simulink model "EMR_vehicle_model_EMRAX188"  (R2023a)
settings: Solver=VariableStepAuto  StartTime=0.0  StopTime=sim_time  RelTol=1e-3
values from neighbouring files (symbols this model uses):
  A_f = 2    [motor_parameters.m]
  air_dens = 1.22521    [motor_parameters.m]
  angle_road = atan(slope_road/100)    [motor_parameters.m]
  C_d = 0.35    [motor_parameters.m]
  converter_efficiency = 0.95    [motor_parameters.m]
  f_r = 0.017    [motor_parameters.m]
  g = 9.8    [motor_parameters.m]
  k_gear = 5    [motor_parameters.m]
  Kantiwind_d = Kp_current_d    [motor_parameters.m]
  Kantiwind_q = Kp_current_q    [motor_parameters.m]
  Ki_current_d = (log(9)/risingtime)*winding_resistance    [motor_parameters.m]
  Ki_current_q = (log(9)/risingtime)*winding_resistance    [motor_parameters.m]
  Kp_current_d = (log(9)/risingtime)*Ld    [motor_parameters.m]
  Kp_current_q = (log(9)/risingtime)*Lq    [motor_parameters.m]
  Kp_speed = m_v/tau_speed    (= 666.666666667)    [motor_parameters.m]
  lambdam = 0.072    [motor_parameters.m]
  Ld = 5.4e-6    (= 5.4e-06)    [motor_parameters.m]
  lower_current_limit = -upper_current_limit    (= -400)    [motor_parameters.m]
  lower_volt_limit = -upper_volt_limit    (= -110)    [motor_parameters.m]
  Lq = 6.0e-6    (= 6e-06)    [motor_parameters.m]
  m_v = 1000    [motor_parameters.m]
  polenumber = 2*polepairs    (= 20)    [motor_parameters.m]
  r_w = 0.26    [motor_parameters.m]
  Rbat = 0.1    [motor_parameters.m]
  upper_current_limit = 400    [motor_parameters.m]
  upper_volt_limit = 110    [motor_parameters.m]
  VDC = 800    [motor_parameters.m]
  wind_speed = 0    [motor_parameters.m]
  winding_resistance = 0.8e-3    (= 0.0008)    [motor_parameters.m]
libraries: simulink x2
settings Model: Creator=citcea  LastModifiedBy=citcea

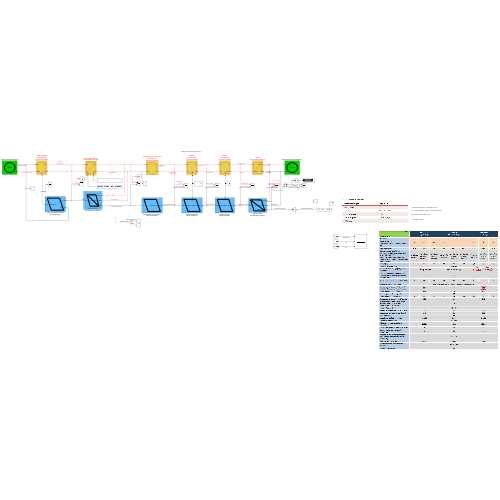
[thumbnail: Simulink's stored preview of the top-level diagram]
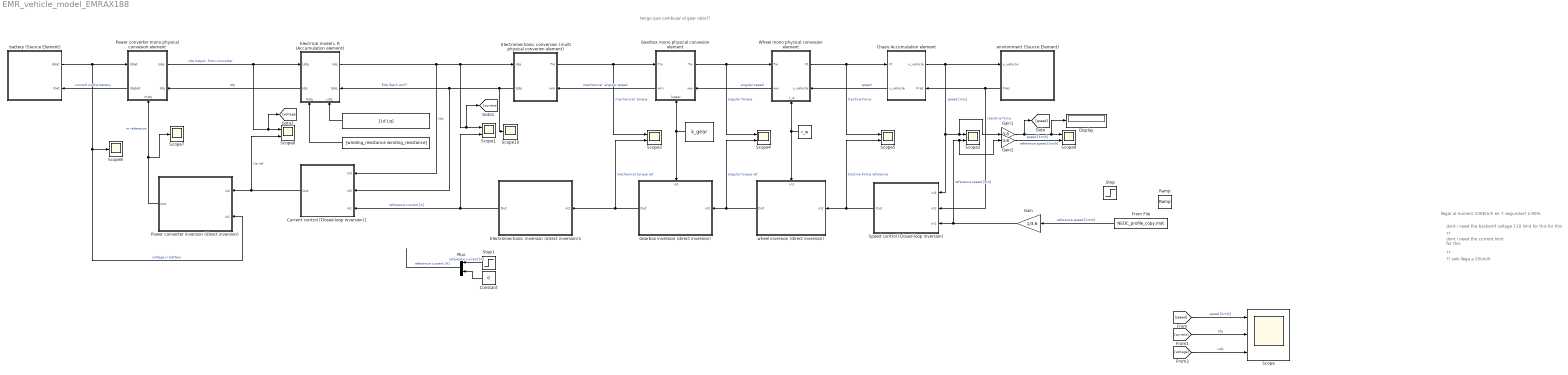
== system EMR_vehicle_model_EMRAX188 ==
  note: dont i need the current limit for this
  note: dont i need the backemf voltage 110 limit for this for this
  note: ?? solo llega a 35km/h
  note: ??
  note: ??
  note: llegar al numero 100Km/h en 7 segundos? o 90%
  note: tengo que cambuiar el gear ratio??
  " " : Constant  Value=[winding_resistance winding_resistance]
  "  " : Constant  Value=k_gear
  "   " : Constant  Value=[Ld Lq]
  "     " : Constant  Value=r_w
  Chasis Accumulation element : Subsystem  mask(CM){}
      settings: LibrarySourceBlock=simulink/REM/EA  PortSchema="{\"entries\":[{\"content\":{\"sides\":[{\"content\":{\"connectorIds\":[\"In1\",\"Out2\"]},\"type\":\"ConnectorPlacement.EquallySpacedRectSide\",\"uuid\":\"dba36025-b2f5-41cb-9761-d1287a9766e1\"},{\"content\":{\"connectorIds\":[\"Out1\",\"In2\"],\"side\":\"RIGHT\"},\"type\":\"ConnectorPlacement.EquallySpacedRectSide\",\"uuid\":\"3ae5e504-7b8f-4c00-bc0d-c89eccd87070\"},{\"content\":{\"side\":\"TOP\"},\"type\":\"ConnectorPlacement.EquallySpacedRectSide\",\"uuid\":\"a4c04bb5-f94e-4b5c-882d-2c32a11c6b0c\"}]},\"type\":\"ConnectorPlacement.EquallySpacedConnector\",\"uuid\":\"0c2b765b-f129-495b-87a6-76b6e14d78ec\"}],\"packageUris\":[\"http://schema.mathworks.com/mf0/Connector/R2020b\"],\"version\":\"1.0\"}"
      mask Display: plot(0,0,100,100,[10,10,90,90,10],[90,10,10,90,90], [10,90],[10,90])
  Constant : Constant  Value=0
  Current control (Closed-loop inversion)1 : Subsystem
      settings: LibrarySourceBlock=|
      | simulink/SMC/Asservissement
      | Correcteur IP
      mask Display: plot(0,0,100,100, [10,30,90,70,10,90],[90,10,10,90,90,10])
  Display : Display
  Electrical model L R (Accumulation element) : Subsystem  mask(CM){}
      settings: LibrarySourceBlock=simulink/REM/EA  PortSchema="{\"entries\":[{\"content\":{\"sides\":[{\"content\":{\"connectorIds\":[\"In1\",\"Out2\"]},\"type\":\"ConnectorPlacement.EquallySpacedRectSide\",\"uuid\":\"eb47d662-bb9b-4acd-af55-2a228b53d8b6\"},{\"content\":{\"connectorIds\":[\"Out1\",\"In4\"],\"side\":\"RIGHT\"},\"type\":\"ConnectorPlacement.EquallySpacedRectSide\",\"uuid\":\"c961b4fe-0170-40df-8b75-bfc3223dfb7e\"},{\"content\":{\"side\":\"TOP\"},\"type\":\"ConnectorPlacement.EquallySpacedRectSide\",\"uuid\":\"6474a77d-3f02-40ef-ac6e-8688b5dfe053\"},{\"content\":{\"connectorIds\":[\"In2\",\"In3\"],\"side\":\"BOTTOM\"},\"type\":\"ConnectorPlacement.EquallySpacedRectSide\",\"uuid\":\"8508c19b-50ed-4acb-b5ce-1a3d4ba68c03\"}]},\"type\":\"ConnectorPlacement.EquallySpacedConnector\",\"uuid\":\"ed0b028c-df9b-42ff-9675-f2eb8371642a\"}],\"packageUris\":[\"http://schema.mathworks.com/mf0/Connector/R2020b\"],\"version\":\"1.0\"}"
      mask Display: plot(0,0,100,100,[10,10,90,90,10],[90,10,10,90,90], [10,90],[10,90])
  Electromechanic conversion (multi physical converion element) : Subsystem
      settings: LibrarySourceBlock=simulink/REM/EC EM  PortSchema="{\"entries\":[{\"content\":{\"sides\":[{\"content\":{\"connectorIds\":[\"In1\",\"Out2\"]},\"type\":\"ConnectorPlacement.EquallySpacedRectSide\",\"uuid\":\"eb47d662-bb9b-4acd-af55-2a228b53d8b6\"},{\"content\":{\"connectorIds\":[\"Out1\",\"In2\"],\"side\":\"RIGHT\"},\"type\":\"ConnectorPlacement.EquallySpacedRectSide\",\"uuid\":\"c961b4fe-0170-40df-8b75-bfc3223dfb7e\"},{\"content\":{\"side\":\"TOP\"},\"type\":\"ConnectorPlacement.EquallySpacedRectSide\",\"uuid\":\"6474a77d-3f02-40ef-ac6e-8688b5dfe053\"},{\"content\":{\"side\":\"BOTTOM\"},\"type\":\"ConnectorPlacement.EquallySpacedRectSide\",\"uuid\":\"5fa3375e-1c74-4447-9856-dc04d4629517\"}]},\"type\":\"ConnectorPlacement.EquallySpacedConnector\",\"uuid\":\"ed0b028c-df9b-42ff-9675-f2eb8371642a\"}],\"packageUris\":[\"http://schema.mathworks.com/mf0/Connector/R2020b\"],\"version\":\"1.0\"}"
      mask Display: plot(0,0,100,100, 1.4*[50,57.68,60.77,63.08,64.97,66.58,68,69.26,70.4, 	71.42,72.36,78.28,80,78.28,72.36,71.42,70.4, 	69.26,68,66.58,64.97,63.08,60.77,57.68,50,42.32, 	39.23,36.92,35.03,33.42,32,30.74,29.6,28.58, 	27.64,21.72,20,21.72,27.64,28.58,29.6,30.74,32, 	33.42,35.03,36.92,39.23,42.32,50]-20, 1.4*[20,21,22,23,24,25,26,27,28,29,30,40,50,60,70,71,72, 	73,74,75,76,77,78,79,80,79,78,77,76,75,74,73,72, 	71,70,60,50,40,30,29,28,27,26,25,24,23,22,21,20]-20)
  Electromechanic inversion (direct inversion)1 : Subsystem
      settings: LibrarySourceBlock=|
      | simulink/SMC/Inversion EC
      | avec mesure
      mask Display: plot(0,0,100,100,[10,30,90,70,10],[90,10,10,90,90])
  From File : FromFile  FileName=NEDC_profile_copy.mat  SampleTime=0
  Gain : Gain  Gain=1/3.6
  Gain1 : Gain  Gain=3.6
  Gain2 : Gain  Gain=3.6
  Gearbox mono physical convesion element : Subsystem  mask(Hacheur){}
      settings: LibrarySourceBlock=simulink/REM/EC Elec  PortSchema="{\"entries\":[{\"content\":{\"sides\":[{\"content\":{\"connectorIds\":[\"In1\",\"Out2\"]},\"type\":\"ConnectorPlacement.EquallySpacedRectSide\",\"uuid\":\"add9fadb-0fb4-43ab-a2d0-7727804eb2c0\"},{\"content\":{\"connectorIds\":[\"Out1\",\"In3\"],\"side\":\"RIGHT\"},\"type\":\"ConnectorPlacement.EquallySpacedRectSide\",\"uuid\":\"87b3f5c0-7da9-421a-ae8a-66afee038ab7\"},{\"content\":{\"side\":\"TOP\"},\"type\":\"ConnectorPlacement.EquallySpacedRectSide\",\"uuid\":\"1a4f8f42-25ac-452e-8ff7-6a9f16bc9892\"},{\"content\":{\"connectorIds\":[\"In2\"],\"side\":\"BOTTOM\"},\"type\":\"ConnectorPlacement.EquallySpacedRectSide\",\"uuid\":\"62447f74-8a92-4f32-9436-8aa69c6390a6\"}]},\"type\":\"ConnectorPlacement.EquallySpacedConnector\",\"uuid\":\"bc965109-6171-440e-b0fd-d7c986fb98ff\"}],\"packageUris\":[\"http://schema.mathworks.com/mf0/Connector/R2020b\"],\"version\":\"1.0\"}"
      mask Display: plot(0,0,100,100,[10,10,90,90,10],[90,10,10,90,90])
  Gearbox inversion (direct inversion) : Subsystem
      settings: PortSchema="{\"entries\":[{\"content\":{\"sides\":[{\"content\":{\"connectorIds\":[\"In1\"]},\"type\":\"ConnectorPlacement.EquallySpacedRectSide\",\"uuid\":\"89460601-ef91-4e28-89d9-1739ebd446c6\"},{\"content\":{\"connectorIds\":[\"Out1\"],\"side\":\"RIGHT\"},\"type\":\"ConnectorPlacement.EquallySpacedRectSide\",\"uuid\":\"1ce34b6b-3a45-4c28-907b-ce0af421135c\"},{\"content\":{\"connectorIds\":[\"In2\"],\"side\":\"TOP\"},\"type\":\"ConnectorPlacement.EquallySpacedRectSide\",\"uuid\":\"71132fa1-5c16-4a2a-8ec5-329f0796b3f7\"}]},\"type\":\"ConnectorPlacement.EquallySpacedConnector\",\"uuid\":\"f923a9d4-f6d6-49f7-92ef-115028220a52\"}],\"packageUris\":[\"http://schema.mathworks.com/mf0/Connector/R2020b\"],\"version\":\"1.0\"}"
      settings: LibrarySourceBlock=|
      | simulink/SMC/Inversion EC
      | avec mesure
      mask Display: plot(0,0,100,100,[10,30,90,70,10],[90,10,10,90,90])
  Mux : Mux  Inputs=2
  Power converter mono physical convesion element : Subsystem  mask(Hacheur){}
      settings: LibrarySourceBlock=simulink/REM/EC Elec  PortSchema="{\"entries\":[{\"content\":{\"sides\":[{\"content\":{\"connectorIds\":[\"In1\",\"Out2\"]},\"type\":\"ConnectorPlacement.EquallySpacedRectSide\",\"uuid\":\"add9fadb-0fb4-43ab-a2d0-7727804eb2c0\"},{\"content\":{\"connectorIds\":[\"Out1\",\"In3\"],\"side\":\"RIGHT\"},\"type\":\"ConnectorPlacement.EquallySpacedRectSide\",\"uuid\":\"87b3f5c0-7da9-421a-ae8a-66afee038ab7\"},{\"content\":{\"side\":\"TOP\"},\"type\":\"ConnectorPlacement.EquallySpacedRectSide\",\"uuid\":\"1a4f8f42-25ac-452e-8ff7-6a9f16bc9892\"},{\"content\":{\"connectorIds\":[\"In2\"],\"side\":\"BOTTOM\"},\"type\":\"ConnectorPlacement.EquallySpacedRectSide\",\"uuid\":\"62447f74-8a92-4f32-9436-8aa69c6390a6\"}]},\"type\":\"ConnectorPlacement.EquallySpacedConnector\",\"uuid\":\"bc965109-6171-440e-b0fd-d7c986fb98ff\"}],\"packageUris\":[\"http://schema.mathworks.com/mf0/Connector/R2020b\"],\"version\":\"1.0\"}"
      mask Display: plot(0,0,100,100,[10,10,90,90,10],[90,10,10,90,90])
  Power converter inversion (direct inversion) : Subsystem
      settings: LibrarySourceBlock=|
      | simulink/SMC/Inversion EC
      | avec mesure
      mask Display: plot(0,0,100,100,[10,30,90,70,10],[90,10,10,90,90])
  Ramp : simulink/Sources/Ramp  slope=100/7  start=0  InitialOutput=0
  Scope : Scope  NumInputPorts=3
  Scope{1..6,9} (7 alike) : Scope  NumInputPorts=2
  Scope10 : Scope
  Scope7 : Scope
  Scope8 : Scope
  Speed control (Closed-loop inversion) : Subsystem
      settings: LibrarySourceBlock=|
      | simulink/SMC/Asservissement
      | Correcteur IP
      mask Display: plot(0,0,100,100, [10,30,90,70,10,90],[90,10,10,90,90,10])
  Step : Step  After=120  SampleTime=0
  Step1 : Step  Time=0  After=100  SampleTime=0
  Wheel mono physical convesion element : Subsystem  mask(Hacheur){}
      settings: LibrarySourceBlock=simulink/REM/EC Elec  PortSchema="{\"entries\":[{\"content\":{\"sides\":[{\"content\":{\"connectorIds\":[\"In1\",\"Out2\"]},\"type\":\"ConnectorPlacement.EquallySpacedRectSide\",\"uuid\":\"add9fadb-0fb4-43ab-a2d0-7727804eb2c0\"},{\"content\":{\"connectorIds\":[\"Out1\",\"In3\"],\"side\":\"RIGHT\"},\"type\":\"ConnectorPlacement.EquallySpacedRectSide\",\"uuid\":\"87b3f5c0-7da9-421a-ae8a-66afee038ab7\"},{\"content\":{\"side\":\"TOP\"},\"type\":\"ConnectorPlacement.EquallySpacedRectSide\",\"uuid\":\"1a4f8f42-25ac-452e-8ff7-6a9f16bc9892\"},{\"content\":{\"connectorIds\":[\"In2\"],\"side\":\"BOTTOM\"},\"type\":\"ConnectorPlacement.EquallySpacedRectSide\",\"uuid\":\"cb138da9-d7db-4398-93fc-4ebc55a3031f\"}]},\"type\":\"ConnectorPlacement.EquallySpacedConnector\",\"uuid\":\"bc965109-6171-440e-b0fd-d7c986fb98ff\"}],\"packageUris\":[\"http://schema.mathworks.com/mf0/Connector/R2020b\"],\"version\":\"1.0\"}"
      mask Display: plot(0,0,100,100,[10,10,90,90,10],[90,10,10,90,90])
  battery (Source Element) : Subsystem
      settings: LibrarySourceBlock=simulink/REM/SE  PortSchema="{\"entries\":[{\"content\":{\"sides\":[{\"content\":{\"connectorIds\":[\"In1\",\"Out1\"]},\"type\":\"ConnectorPlacement.EquallySpacedRectSide\",\"uuid\":\"5172ac9f-d5c1-4cd8-b96a-59474b42a5b1\"},{\"content\":{\"side\":\"RIGHT\"},\"type\":\"ConnectorPlacement.EquallySpacedRectSide\",\"uuid\":\"2f1e5561-012a-4a4f-9618-a2ea7815b4bb\"},{\"content\":{\"side\":\"TOP\"},\"type\":\"ConnectorPlacement.EquallySpacedRectSide\",\"uuid\":\"04863bbd-e2a6-484f-917f-c8a12d5dbdba\"}]},\"type\":\"ConnectorPlacement.EquallySpacedConnector\",\"uuid\":\"d1a021b9-616a-4321-9b00-fb5e0223e97f\"}],\"packageUris\":[\"http://schema.mathworks.com/mf0/Connector/R2020b\"],\"version\":\"1.0\"}"
      mask Display:
      | plot(0,0,100,100, 1.2*[50,57.68,60.77,63.08,64.97,66.58,68,69.26,70.4, 	71.42,72.36,78.28,80,78.28,72.36,71.42,70.4, 	69.26,68,66.58,64.97,63.08,60.77,57.68,50,42.32, 	39.23,36.92,35.03,33.42,32,30.74,29.6,28.58, 	27.64,21.72,20,21.72,27.64,28.58,29.6,30.74,32, 	33.42,35.03,36.92,39.23,42.32,50]-10, 1.2*[20,21,22,23,24,25,26,27,28,29,30,40,50,60,70,71,72, 	73,74,75,76,77,78,79,80,79,78,77,76,75,74,73,72, 	71,70,60,50,40,30,29,28,27,26,25,24,23,22,21,20]-10)
      | disp('Source')
  environment (Source Element) : Subsystem
      settings: LibrarySourceBlock=simulink/REM/SE  PortSchema="{\"entries\":[{\"content\":{\"sides\":[{\"content\":{\"connectorIds\":[\"In1\",\"Out1\"]},\"type\":\"ConnectorPlacement.EquallySpacedRectSide\",\"uuid\":\"5172ac9f-d5c1-4cd8-b96a-59474b42a5b1\"},{\"content\":{\"side\":\"RIGHT\"},\"type\":\"ConnectorPlacement.EquallySpacedRectSide\",\"uuid\":\"2f1e5561-012a-4a4f-9618-a2ea7815b4bb\"},{\"content\":{\"side\":\"TOP\"},\"type\":\"ConnectorPlacement.EquallySpacedRectSide\",\"uuid\":\"04863bbd-e2a6-484f-917f-c8a12d5dbdba\"}]},\"type\":\"ConnectorPlacement.EquallySpacedConnector\",\"uuid\":\"d1a021b9-616a-4321-9b00-fb5e0223e97f\"}],\"packageUris\":[\"http://schema.mathworks.com/mf0/Connector/R2020b\"],\"version\":\"1.0\"}"
      mask Display:
      | plot(0,0,100,100, 1.2*[50,57.68,60.77,63.08,64.97,66.58,68,69.26,70.4, 	71.42,72.36,78.28,80,78.28,72.36,71.42,70.4, 	69.26,68,66.58,64.97,63.08,60.77,57.68,50,42.32, 	39.23,36.92,35.03,33.42,32,30.74,29.6,28.58, 	27.64,21.72,20,21.72,27.64,28.58,29.6,30.74,32, 	33.42,35.03,36.92,39.23,42.32,50]-10, 1.2*[20,21,22,23,24,25,26,27,28,29,30,40,50,60,70,71,72, 	73,74,75,76,77,78,79,80,79,78,77,76,75,74,73,72, 	71,70,60,50,40,30,29,28,27,26,25,24,23,22,21,20]-10)
      | disp('Source')
  wheel inversion (direct inversion) : Subsystem
      settings: PortSchema="{\"entries\":[{\"content\":{\"sides\":[{\"content\":{\"connectorIds\":[\"In1\"]},\"type\":\"ConnectorPlacement.EquallySpacedRectSide\",\"uuid\":\"89460601-ef91-4e28-89d9-1739ebd446c6\"},{\"content\":{\"connectorIds\":[\"Out1\"],\"side\":\"RIGHT\"},\"type\":\"ConnectorPlacement.EquallySpacedRectSide\",\"uuid\":\"1ce34b6b-3a45-4c28-907b-ce0af421135c\"},{\"content\":{\"connectorIds\":[\"In2\"],\"side\":\"TOP\"},\"type\":\"ConnectorPlacement.EquallySpacedRectSide\",\"uuid\":\"71132fa1-5c16-4a2a-8ec5-329f0796b3f7\"}]},\"type\":\"ConnectorPlacement.EquallySpacedConnector\",\"uuid\":\"f923a9d4-f6d6-49f7-92ef-115028220a52\"}],\"packageUris\":[\"http://schema.mathworks.com/mf0/Connector/R2020b\"],\"version\":\"1.0\"}"
      settings: LibrarySourceBlock=|
      | simulink/SMC/Inversion EC
      | avec mesure
      mask Display: plot(0,0,100,100,[10,30,90,70,10],[90,10,10,90,90])
  wires:
  environment (Source Element)/1(Fres) -> Chasis Accumulation element/2(Fres), Speed control (Closed-loop inversion)/2(in2)  "resistive force"
  Speed control (Closed-loop inversion)/1(Out) -> Scope5/2, wheel inversion (direct inversion)/1(in2)  "tractive Force reference"
  Chasis Accumulation element/2(v_vehicle) -> Wheel mono physical convesion element/3(v_vehicle)  "speed"
  "     "/1 -> Wheel mono physical convesion element/2(r_w), wheel inversion (direct inversion)/2(in1)
  Gearbox mono physical convesion element/1("Tw ") -> Scope4/1, Wheel mono physical convesion element/1(Tw)  "angular Torque"
  Wheel mono physical convesion element/2(ww) -> Gearbox mono physical convesion element/3(ww)  "angular speed"
  "  "/1 -> Gearbox inversion (direct inversion)/2(in1), Gearbox mono physical convesion element/2(kgear)
  Electromechanic conversion (multi physical converion element)/1("Tm ") -> Scope3/1, Gearbox mono physical convesion element/1(Tm)  "mechanical  torque"
  Gearbox mono physical convesion element/2(wm) -> Electromechanic conversion (multi physical converion element)/2(wm)  "mechanical  angular speed"
  Electrical model L R (Accumulation element)/1("Idq ") -> Current control (Closed-loop inversion)1/1(in3), [current], Scope1/1, Electromechanic conversion (multi physical converion element)/1(Idq)  "Idq"
  Electromechanic conversion (multi physical converion element)/2(Edq) -> Scope10/1, Current control (Closed-loop inversion)1/2(in5), Electrical model L R (Accumulation element)/4(Edq)  "Edq (back emf)"
  Electrical model L R (Accumulation element)/2(Idq) -> Power converter mono physical convesion element/3(Idq)  "Idq"
  Power converter mono physical convesion element/1("Udq ") -> Electrical model L R (Accumulation element)/1(Udq), [voltage], Scope6/1  "vdq output  from converter"
  Power converter mono physical convesion element/2("Idqbat  ") -> battery (Source Element)/1(Ibat)  "current on the battery"
  battery (Source Element)/1(Ubat) -> Power converter inversion (direct inversion)/2(in1), Scope8/1, Power converter mono physical convesion element/1(Ubat)  "voltage in battery"
  " "/1 -> Electrical model L R (Accumulation element)/2(Rdq)
  "   "/1 -> Electrical model L R (Accumulation element)/3(Ldq)
  Chasis Accumulation element/1("v_vehicle ") -> Speed control (Closed-loop inversion)/1(in3), Gain1/1, Scope2/1, environment (Source Element)/1(v_vehicle)  "speed [m/s]"
  wheel inversion (direct inversion)/1(Out) -> Gearbox inversion (direct inversion)/1(in2), Scope4/2  "angular torque ref"
  Gearbox inversion (direct inversion)/1(Out) -> Scope3/2, Electromechanic inversion (direct inversion)1/1(in2)  "mechanical torque ref"
  Current control (Closed-loop inversion)1/1(Out) -> Scope6/2, Power converter inversion (direct inversion)/1(in2)  "Ua ref"
  Power converter inversion (direct inversion)/1(Out) -> Scope7/1, Power converter mono physical convesion element/2(mdq)  "m reference"
  Gain/1 -> Gain2/1, Scope2/2, Speed control (Closed-loop inversion)/3(in1)  "reference speed [m/s]"
  From File/1 -> Gain/1  "reference speed [km/h]"
  Gain2/1 -> Scope9/2  "reference speed [km/h]"
  Gain1/1 -> [speed], Display/1, Scope9/1  "speed [km/h]"
  Electromechanic inversion (direct inversion)1/1(Out) -> Current control (Closed-loop inversion)1/3(in1), Scope1/2  "reference current [A]"
  Wheel mono physical convesion element/1("Ft ") -> Chasis Accumulation element/1(Ft), Scope5/1  "tractive Force"
  Step1/1 -> Mux/1  "reference current [A]"
  Constant/1 -> Mux/2
  Mux/1 -> ?  "reference current [A]"
  [speed] -> Scope/1  "speed [km/h]"
  [current] -> Scope/2  "Idq"
  [voltage] -> Scope/3  "vdq"

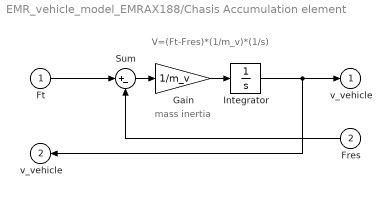
== system EMR_vehicle_model_EMRAX188/Chasis Accumulation element ==
  note: V=(Ft-Fres)*(1/m_v)*(1/s)
  note: mass inertia
  Ft : Inport
  Fres : Inport  Port=2
  Gain : Gain  Gain=1/m_v
  Integrator : Integrator
  Sum : Sum  Inputs=|+-
  "v_vehicle " : Outport  InitialOutput=0
  v_vehicle : Outport  Port=2  InitialOutput=0
  wires:
  Gain/1 -> Integrator/1
  Sum/1 -> Gain/1
  Integrator/1 -> v_vehicle/1, "v_vehicle "/1
  Ft/1 -> Sum/1
  Fres/1 -> Sum/2

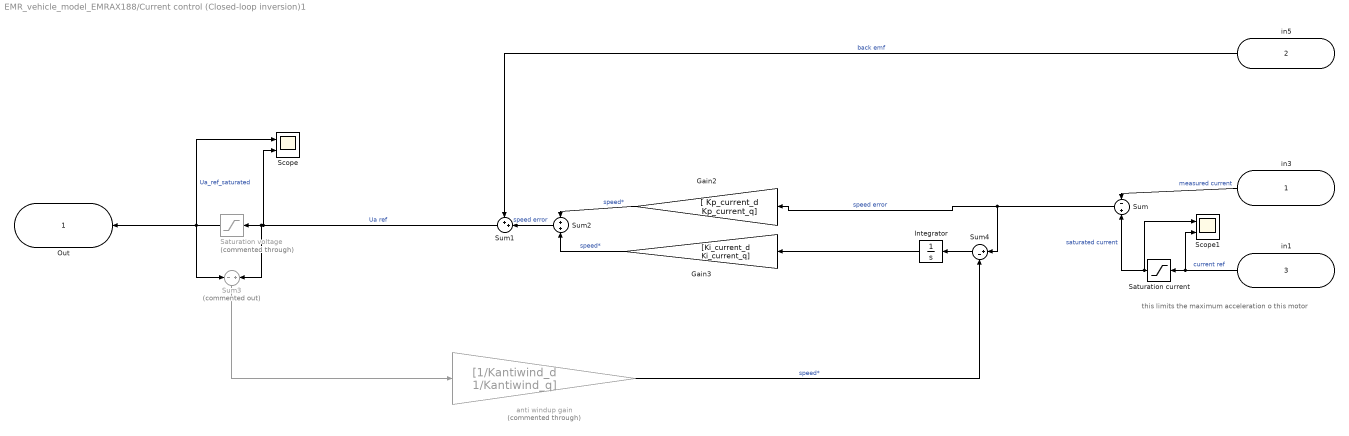
== system EMR_vehicle_model_EMRAX188/Current control (Closed-loop inversion)1 ==
  note: this limits the maximum acceleration o this motor
  in3 : Inport
  in5 : Inport  Port=2
  in1 : Inport  Port=3
  Gain2 : Gain  Gain=[ Kp_current_d Kp_current_q]
  Gain3 : Gain  Gain=[Ki_current_d Ki_current_q]
  Integrator : Integrator
  Saturation current : Saturate  UpperLimit=upper_current_limit  LowerLimit=lower_current_limit
  Saturation voltage : Saturate  Commented=through  UpperLimit=upper_volt_limit  LowerLimit=lower_volt_limit
  Scope : Scope  NumInputPorts=2
  Scope1 : Scope  NumInputPorts=2
  Sum : Sum  Inputs=-+
  Sum1 : Sum  Inputs=++|
  Sum2 : Sum
  Sum3 : Sum  Commented=on  Inputs=-|+
  Sum4 : Sum  Inputs=|+-
  anti windup gain : Gain  Commented=through  Gain=[1/Kantiwind_d 1/Kantiwind_q]
  Out : Outport  InitialOutput=0
  wires:
  in3/1 -> Sum/1  "measured current"
  in1/1 -> Scope1/2, Saturation current/1  "current ref"
  Sum1/1 -> Sum3/2, Saturation voltage/1, Scope/2  "Ua ref"
  Sum/1 -> Gain2/1, Sum4/1  "speed error"
  Gain2/1 -> Sum2/1  "speed*"
  in5/1 -> Sum1/1  "back emf"
  Gain3/1 -> Sum2/2  "speed*"
  Sum2/1 -> Sum1/2  "speed error"
  Integrator/1 -> Gain3/1
  Saturation current/1 -> Sum/2, Scope1/1  "saturated current"
  Saturation voltage/1 -> Sum3/1, Scope/1, Out/1  "Ua_ref_saturated"
  Sum3/1 -> anti windup gain/1
  anti windup gain/1 -> Sum4/2  "speed*"
  Sum4/1 -> Integrator/1

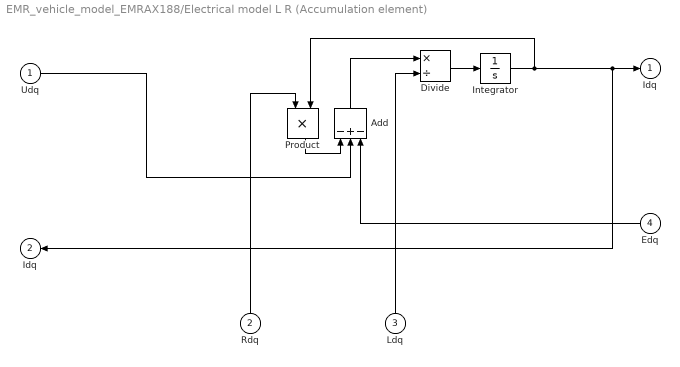
== system EMR_vehicle_model_EMRAX188/Electrical model L R (Accumulation element) ==
  Udq : Inport
  Rdq : Inport  Port=2
  Ldq : Inport  Port=3
  Edq : Inport  Port=4
  Add : Sum  Inputs=-+-
  Divide : Product  Inputs=*/
  Integrator : Integrator
  Product : Product
  "Idq " : Outport  InitialOutput=0
  Idq : Outport  Port=2  InitialOutput=0
  wires:
  Edq/1 -> Add/3
  Udq/1 -> Add/2
  Integrator/1 -> Product/2, "Idq "/1, Idq/1
  Add/1 -> Divide/1
  Ldq/1 -> Divide/2
  Divide/1 -> Integrator/1
  Product/1 -> Add/1
  Rdq/1 -> Product/1

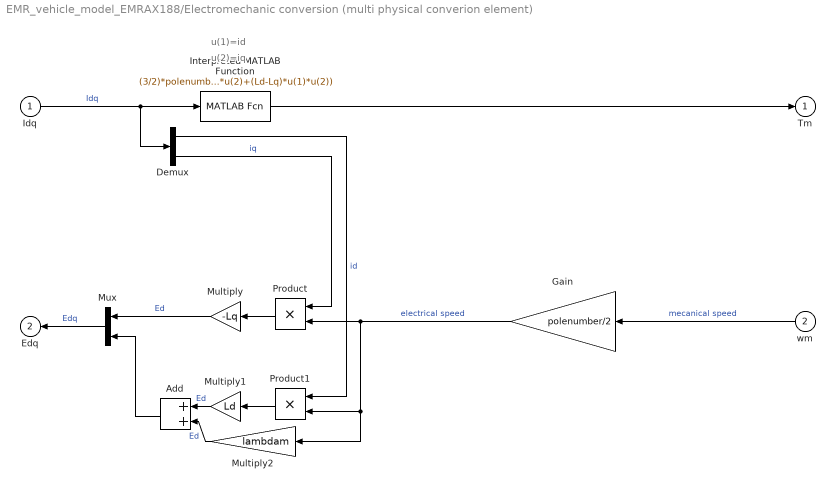
== system EMR_vehicle_model_EMRAX188/Electromechanic conversion (multi physical converion element) ==
  note: u(1)=id
  note: u(2)=iq
  Idq : Inport
  wm : Inport  Port=2
  Add : Sum
  Demux : Demux  Outputs=2
  Gain : Gain  Gain=polenumber/2
  Interpreted MATLAB Function : MATLABFcn  MATLABFcn=(3/2)*polenumber/2*(lambdam*u(2)+(Ld-Lq)*u(1)*u(2))  OutputDimensions=1
  Multiply : Gain  Gain=-Lq
  Multiply1 : Gain  Gain=Ld
  Multiply2 : Gain  Gain=lambdam
  Mux : Mux  Inputs=2
  Product : Product
  Product1 : Product
  "Tm " : Outport  InitialOutput=0
  Edq : Outport  Port=2  InitialOutput=0
  wires:
  Idq/1 -> Demux/1, Interpreted MATLAB Function/1  "Idq"
  Interpreted MATLAB Function/1 -> "Tm "/1
  wm/1 -> Gain/1  "mecanical speed"
  Demux/1 -> Product1/1  "id"
  Demux/2 -> Product/1  "iq"
  Mux/1 -> Edq/1  "Edq"
  Gain/1 -> Multiply2/1, Product1/2, Product/2  "electrical speed"
  Product/1 -> Multiply/1
  Multiply/1 -> Mux/1  "Ed"
  Product1/1 -> Multiply1/1
  Multiply1/1 -> Add/1  "Ed"
  Add/1 -> Mux/2
  Multiply2/1 -> Add/2  "Ed"

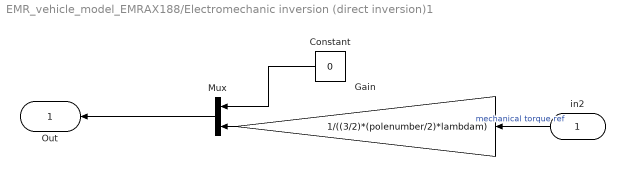
== system EMR_vehicle_model_EMRAX188/Electromechanic inversion (direct inversion)1 ==
  in2 : Inport
  Constant : Constant  Value=0
  Gain : Gain  Gain=1/((3/2)*(polenumber/2)*lambdam)
  Mux : Mux  Inputs=2
  Out : Outport  InitialOutput=0
  wires:
  Mux/1 -> Out/1
  Gain/1 -> Mux/2
  in2/1 -> Gain/1  "mechanical torque ref"
  Constant/1 -> Mux/1

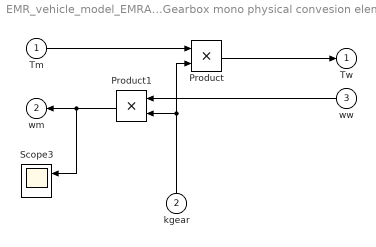
== system EMR_vehicle_model_EMRAX188/Gearbox mono physical convesion element ==
  Tm : Inport
  kgear : Inport  Port=2
  ww : Inport  Port=3
  Product : Product
  Product1 : Product
  Scope3 : Scope  NumInputPorts=2
  "Tw " : Outport  InitialOutput=0
  wm : Outport  Port=2  InitialOutput=0
  wires:
  Product1/1 -> Scope3/1, wm/1
  kgear/1 -> Product1/2, Product/2
  ww/1 -> Product1/1
  Product/1 -> "Tw "/1
  Tm/1 -> Product/1

== system EMR_vehicle_model_EMRAX188/Gearbox inversion (direct inversion) ==
  in2 : Inport
  in1 : Inport  Port=2
  Divide : Product  Inputs=/*
  Out : Outport  InitialOutput=0
  wires:
  Divide/1 -> Out/1  "mecanical torque"
  in2/1 -> Divide/2  "angular torque ref"
  in1/1 -> Divide/1  "k gear"

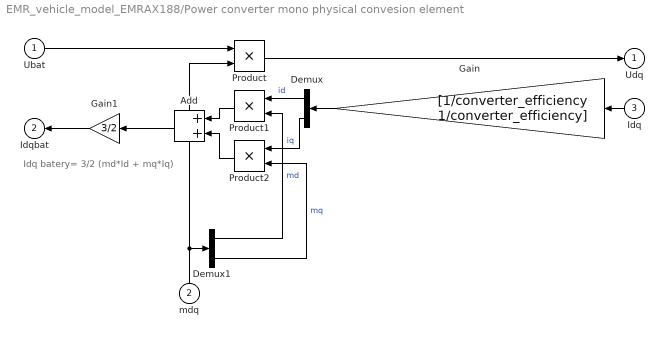
== system EMR_vehicle_model_EMRAX188/Power converter mono physical convesion element ==
  note: Idq batery= 3/2 (md*Id + mq*Iq)
  Ubat : Inport
  mdq : Inport  Port=2
  Idq : Inport  Port=3
  Add : Sum
  Demux : Demux  Outputs=2
  Demux1 : Demux  Outputs=2
  Gain : Gain  Gain=[1/converter_efficiency 1/converter_efficiency]
  Gain1 : Gain  Gain=3/2
  Product : Product
  Product1 : Product
  Product2 : Product
  "Udq " : Outport  InitialOutput=0
  "Idqbat  " : Outport  Port=2  InitialOutput=0
  wires:
  Idq/1 -> Gain/1
  Ubat/1 -> Product/1
  mdq/1 -> Demux1/1, Product/2
  Product/1 -> "Udq "/1
  Gain/1 -> Demux/1
  Gain1/1 -> "Idqbat  "/1
  Demux/1 -> Product1/1  "id"
  Demux/2 -> Product2/1  "iq"
  Demux1/1 -> Product1/2  "md"
  Demux1/2 -> Product2/2  "mq"
  Product1/1 -> Add/1
  Product2/1 -> Add/2
  Add/1 -> Gain1/1

== system EMR_vehicle_model_EMRAX188/Power converter inversion (direct inversion) ==
  in2 : Inport
  in1 : Inport  Port=2
  Divide : Product  Inputs=/*
  Saturation m ( we got regenerative braking) : Saturate  UpperLimit=1  LowerLimit=-1
  Out : Outport  InitialOutput=0
  wires:
  Divide/1 -> Saturation m ( we got regenerative braking)/1  "m_not saturated"
  in2/1 -> Divide/2  "Ua_dq ref"
  in1/1 -> Divide/1  "Ubat_dq"
  Saturation m ( we got regenerative braking)/1 -> Out/1  "mdq_ref_saturated"

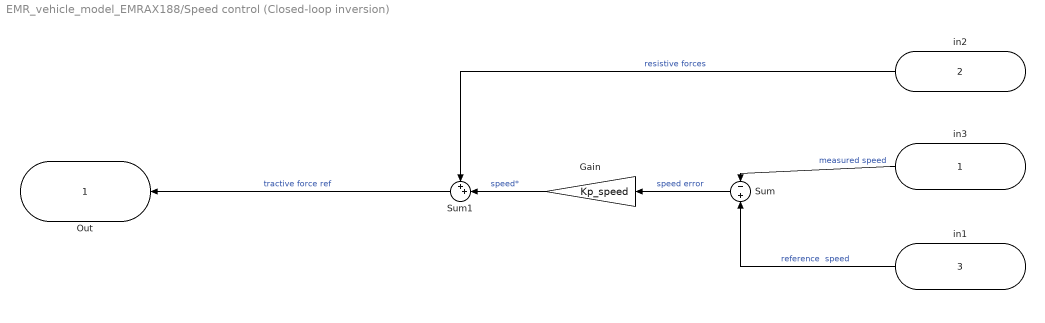
== system EMR_vehicle_model_EMRAX188/Speed control (Closed-loop inversion) ==
  in3 : Inport
  in2 : Inport  Port=2
  in1 : Inport  Port=3
  Gain : Gain  Gain=Kp_speed
  Sum : Sum  Inputs=-+
  Sum1 : Sum  Inputs=++|
  Out : Outport  InitialOutput=0
  wires:
  in3/1 -> Sum/1  "measured speed"
  in1/1 -> Sum/2  "reference  speed"
  Sum1/1 -> Out/1  "tractive force ref"
  Sum/1 -> Gain/1  "speed error"
  Gain/1 -> Sum1/2  "speed*"
  in2/1 -> Sum1/1  "resistive forces"

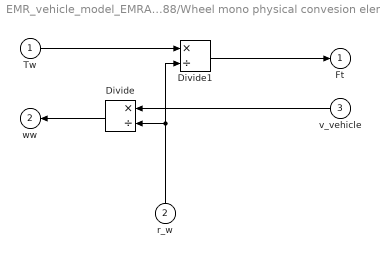
== system EMR_vehicle_model_EMRAX188/Wheel mono physical convesion element ==
  Tw : Inport
  r_w : Inport  Port=2
  v_vehicle : Inport  Port=3
  Divide : Product  Inputs=*/
  Divide1 : Product  Inputs=*/
  "Ft " : Outport  InitialOutput=0
  ww : Outport  Port=2  InitialOutput=0
  wires:
  Divide/1 -> ww/1
  v_vehicle/1 -> Divide/1
  r_w/1 -> Divide1/2, Divide/2
  Divide1/1 -> "Ft "/1
  Tw/1 -> Divide1/1

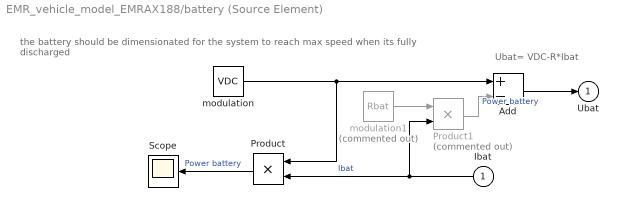
== system EMR_vehicle_model_EMRAX188/battery (Source Element) ==
  note: the battery should be dimensionated for the system to reach
      | max speed when its fully discharged
  note: Ubat= VDC-R*Ibat
  Ibat : Inport
  Add : Sum  Inputs=+-
  Product : Product
  Product1 : Product  Commented=on
  Scope : Scope
  modulation : Constant  Value=VDC
  modulation1 : Constant  Commented=on  Value=Rbat
  Ubat : Outport  InitialOutput=0
  wires:
  modulation/1 -> Add/1, Product/1
  Ibat/1 -> Product1/2, Product/2  "Ibat"
  Product/1 -> Scope/1  "Power battery"
  Add/1 -> Ubat/1
  Product1/1 -> Add/2  "Power battery"
  modulation1/1 -> Product1/1

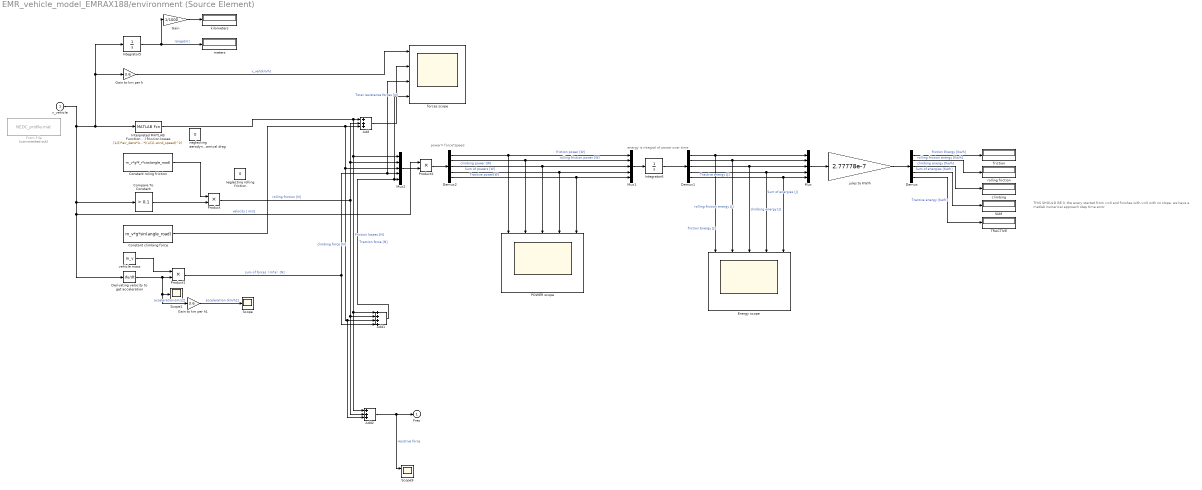
== system EMR_vehicle_model_EMRAX188/environment (Source Element) ==
  note: energy is integral of power over time
  note: power= force*speed
  note: THIS SHOULD BE 0, the enery started from v=0 and finishes with v=0 with no slope. we have a matlab numerical approach step time error
  v_vehicle : Inport
  Add : Sum  Inputs=+++
  Add1 : Sum  Inputs=++++
  Add2 : Sum  Inputs=+++
  Compare To Constant : simulink/Logic and Bit Operations/Compare To Constant  relop=>  const=0.1  OutDataTypeStr=boolean  ZeroCross=off
  Constant climbing force : Constant  Value=m_v*g*sin(angle_road)
  Constant roling friction : Constant  Value=m_v*g*f_r*cos(angle_road)
  Demux : Demux  Outputs=5
  Demux1 : Demux  Outputs=5
  Demux2 : Demux  Outputs=5
  Derivating velocity to get acceleration : Derivative
  Energy scope : Scope  NumInputPorts=5
  From File : FromFile  Commented=on  FileName=NEDC_profile.mat  SampleTime=0
  Gain : Gain  Gain=1/1000
  Gain to km per h : Gain  Gain=3.6
  Gain to km per h1 : Gain  Gain=3.6
  Integrator5 : Integrator
  Integrator6 : Integrator
  Interpreted MATLAB Function Aerodinamical friccion losses : MATLABFcn  MATLABFcn=(1/2)*air_dens*A_f*C_d*((u(1)-wind_speed)^2)
  Mux : Mux  Inputs=5
  Mux1 : Mux  Inputs=5
  Mux2 : Mux  Inputs=5
  POWER scope : Scope  NumInputPorts=5
  Product : Product
  Product1 : Product
  Product2 : Product
  "SUM " : Display
  Scope : Scope
  Scope1 : Scope
  Scope9 : Scope  NumInputPorts=2
  TRACTIVE : Display
  climbing : Display
  forces scope : Scope  NumInputPorts=4
  friction : Display
  jules to KW/h : Gain  Gain=2.77778e-7
  kilometers : Display
  meters : Display
  neglecting aerodynamical drag : Constant  Value=0
  neglecting rolling friction : Constant  Value=0
  "rolling friction " : Display
  vehicle mass : Constant  Value=m_v
  Fres : Outport  InitialOutput=0
  wires:
  Gain/1 -> kilometers/1
  v_vehicle/1 -> Derivating velocity to get acceleration/1, Product2/1, Compare To Constant/1, Integrator5/1, Gain to km per h/1, Interpreted MATLAB Function Aerodinamical friccion losses/1  "velocity [ m/s]"
  Add1/1 -> forces scope/4, Mux2/5  "Traction force [N]"
  Demux2/2 -> Mux1/2, POWER scope/2  "rolling friction power [W]"
  Integrator5/1 -> Gain/1, meters/1  "range[m]"
  Demux/3 -> climbing/1  "climbing energy [Kw/h]"
  Constant roling friction/1 -> Product/1
  Mux2/1 -> Product2/2
  Gain to km per h/1 -> forces scope/1  "v_veh[km/h]"
  Demux1/3 -> Energy scope/3, Mux/3  "climbing energy [J]"
  Compare To Constant/1 -> Product/2
  Demux2/5 -> Mux1/5, POWER scope/5  "Tractive power[W]"
  Mux1/1 -> Integrator6/1
  Product2/1 -> Demux2/1
  jules to KW/h/1 -> Demux/1
  Demux1/2 -> Energy scope/2, Mux/2  "rolling friction energy [J]"
  Demux/2 -> "rolling friction "/1  "rolling friction energy [Kw/h]"
  Demux2/1 -> Mux1/1, POWER scope/1  "friction power [W]"
  Constant climbing force/1 -> Add2/3, Add1/3, Mux2/3, Add/3  "climbing force [N]"
  Add/1 -> forces scope/2  "Total resistance forces [N]"
  Interpreted MATLAB Function Aerodinamical friccion losses/1 -> Add1/1, Add2/1, Mux2/1, Add/1  "Friction losses [N]"
  Demux2/4 -> Mux1/4, POWER scope/4  "Sum of powers [W]"
  Demux1/4 -> Energy scope/4, Mux/4  "Sum of energies [J]"
  Demux1/1 -> Mux/1, Energy scope/1  "friction Energy [J]"
  Demux1/5 -> Energy scope/5, Mux/5  "Tractive energy [J]"
  Derivating velocity to get acceleration/1 -> Scope1/1, Gain to km per h1/1, Product1/2  "acceleration [m/s2]"
  Integrator6/1 -> Demux1/1
  Mux/1 -> jules to KW/h/1
  Demux2/3 -> Mux1/3, POWER scope/3  "climbing power [W]"
  Product/1 -> Add/2, Mux2/2, Add2/2, Add1/2  "rolling friction [N]"
  Demux/5 -> TRACTIVE/1  "Tractive energy [Kw/h]"
  vehicle mass/1 -> Product1/1
  Demux/4 -> "SUM "/1  "Sum of energies [Kw/h]"
  Demux/1 -> friction/1  "friction Energy [Kw/h]"
  Product1/1 -> Mux2/4, forces scope/3, Add1/4  "sum of forces  (m*a)  [N]"
  Gain to km per h1/1 -> Scope/1  "acceleration [km/h2]"
  Add2/1 -> Scope9/1, Fres/1  "resistive force"

== system EMR_vehicle_model_EMRAX188/wheel inversion (direct inversion) ==
  in2 : Inport
  in1 : Inport  Port=2
  Product : Product
  Out : Outport  InitialOutput=0
  wires:
  Product/1 -> Out/1  "angular torque ref"
  in2/1 -> Product/2  "tractive torque ref"
  in1/1 -> Product/1  "r_w"
